simulink model "DirectedEvent5"  (R2020b)
settings: Solver=VariableStepAuto  StartTime=0.0  StopTime=0.1  RelTol=1e-3
settings Model: Creator=86188  LastModifiedBy=apple
settings DataIOCC: ReturnWorkspaceOutputs=off
settings DebuggingCC: ArithmeticOperatorsInVariantConditions=warning
settings SFSimCC: SimUseLocalCustomCode=off  CustomCodeUndefinedFunction=UseInterfaceOnly
settings RTWCC: RTWUseLocalCustomCode=off

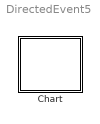
== system DirectedEvent5 ==
  Chart : Stateflow chart  TreatAsAtomicUnit=on

== stateflow chart DirectedEvent5/Chart ==
  settings: updateMethod=DISCRETE  sampleTime=0.1
  state AM
    state A [parallel]
      settings: executionOrder=1
      state A2
        en: fprintf("en_A2")
        ex: fprintf("ex_A2")
      state A1
        en: fprintf("en_A1")
        ex: fprintf("ex_A1")
      (default) -> A1
      A1 -> A2 : [data==1]{send(E_one, AM.B.B1.B2)}
      A2 -> A1 : E_two
    state B [parallel]
      settings: executionOrder=2
      state B1
        state B2
          en: fprintf("en_B2")
          ex: fprintf("ex_B2")
          state B21
            en: fprintf("en_B21")
            ex: fprintf("ex_B21")
          state B22
            en: fprintf("en_B22")
            ex: fprintf("ex_B22")
          (default) -> B21
          B21 -> B22 : E_one
        state B3
          en: fprintf("en_B2")
          ex: fprintf("ex_B2")
        (default) -> B2
        B2 -> B3 : E_two
        B3 -> B2 : E_one
      state B4
        en: fprintf("en_B4")
        ex: fprintf("ex_B4")
      (default) -> B1
      B1 -> B4 : E_one
      B4 -> B1 : E_two
  (default) -> AM : {data = 1;}
  data: data local =1
  events: E_one local FUNCTION_CALL_EVENT; E_two local FUNCTION_CALL_EVENT
